simulink model "buck_hysteresis"  (Simulink 8.9)
settings: Solver=ode45  StartTime=0.0  StopTime=Tmax  RelTol=1e-3  EnableMultiTasking=on
values from neighbouring files (symbols this model uses):
  a00c = sys(1).Ac(1,1)    [buck_parameters.m]
  a00d = sys(1).Ad(1,1)    [buck_parameters.m]
  a00o = sys(1).Ao(1,1)    [buck_parameters.m]
  a01c = sys(1).Ac(1,2)    [buck_parameters.m]
  a01d = sys(1).Ad(1,2)    [buck_parameters.m]
  a01o = sys(1).Ao(1,2)    [buck_parameters.m]
  a10c = sys(1).Ac(2,1)    [buck_parameters.m]
  a10d = sys(1).Ad(2,1)    [buck_parameters.m]
  a10o = sys(1).Ao(2,1)    [buck_parameters.m]
  a11c = sys(1).Ac(2,2)    [buck_parameters.m]
  a11d = sys(1).Ad(2,2)    [buck_parameters.m]
  a11o = sys(1).Ao(2,2)    [buck_parameters.m]
  b0c = sys(1).Bc(1)    [buck_parameters.m]
  b0d = sys(1).Bd(1)    [buck_parameters.m]
  b0o = sys(1).Bo(1)    [buck_parameters.m]
  b1c = sys(1).Bc(2)    [buck_parameters.m]
  b1d = sys(1).Bd(2)    [buck_parameters.m]
  b1o = sys(1).Bo(2)    [buck_parameters.m]
  i0 = 0    [buck_parameters.m]
  v0 = 0    [buck_parameters.m]
  Vref = 12    [buck_parameters.m]
  Vtol = Vref/120    (= 0.1)    [buck_parameters.m]
settings Model: Creator=Omar Ali Beg  LastModifiedBy=LuanNguyen
settings OptimizationCC: ExpressionDepthLimit=2147483647
settings DebuggingCC: MaxConsecutiveZCsMsg=none  MultiTaskDSMMsg=warning  MultiTaskCondExecSysMsg=none  FcnCallInpInsideContextMsg=error  StrictBusMsg=None
settings GRTTargetCC: CombineOutputUpdateFcns=on  GRTInterface=off

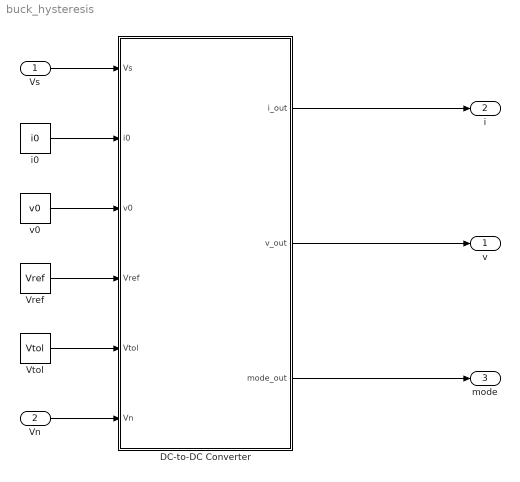
== system buck_hysteresis ==
  Vs : Inport
  Vn : Inport  Port=2
  DC-to-DC Converter : Stateflow chart  TreatAsAtomicUnit=on
  Vref : Constant  Value=Vref
  Vtol : Constant  Value=Vtol
  i0 : Constant  Value=i0
  v0 : Constant  Value=v0
  v : Outport
  i : Outport  Port=2
  mode : Outport  Port=3
  wires:
  DC-to-DC Converter/2(v_out) -> v/1
  Vs/1 -> DC-to-DC Converter/1(Vs)
  i0/1 -> DC-to-DC Converter/2(i0)
  v0/1 -> DC-to-DC Converter/3(v0)
  Vref/1 -> DC-to-DC Converter/4(Vref)
  DC-to-DC Converter/3(mode_out) -> mode/1
  Vtol/1 -> DC-to-DC Converter/5(Vtol)
  DC-to-DC Converter/1(i_out) -> i/1
  Vn/1 -> DC-to-DC Converter/6(Vn)

== stateflow chart DC-to-DC Converter ==
  settings: updateMethod=CONTINUOUS
  state Discontinuous
    du:
    i_dot = a00d*i+a01d*v+b0d*(Vs+Vn);
    v_dot = a10d*i+a11d*v+b1d*(Vs+Vn);
    t_dot = 1;
    i_out =i;
    v_out = v;
    mode_out=3;
  state Charging
    du:
    i_dot = a00c*i+a01c*v+b0c*(Vs+Vn);
    v_dot = a10c*i+a11c*v+b1c*(Vs+Vn);
    t_dot = 1;
    i_out = i;
    v_out = v;
    mode_out=2;
  state Discharging
    du:
    i_dot = a00o*i+a01o*v+b0o*(Vs+Vn);
    v_dot = a10o*i+a11o*v+b1o*(Vs+Vn);
    t_dot = 1;
    i_out = i;
    v_out = v;
    mode_out=1;
  Discontinuous -> Charging : [v <= Vref-Vtol]
  Discharging -> Discontinuous [order 1] : [i <= 0]
  (default) -> Charging : {i = i0;
      | v = v0;}
  Charging -> Discharging : [v >= Vref+Vtol]
  Discharging -> Charging [order 2] : [v <= Vref-Vtol]
  data: t local double; i_out output double; v_out output double; i local double; a00o local double; Vs input double =120; a01o local double; a10o local double; a11o local double; a00c local double; a01c local double; a10c local double; a11c local double; b0o local double; b1o local double; b0c local double; b1c local double; v local double; i0 input double; v0 input double; a01d local double; a10d local double; a11d local double; a00d local double; b0d local double; b1d local double; Vref input double =120; mode_out output double; Vtol input double =120; Vn input double =120
  data t settings: updateMethod=SF_CONTINUOUS_TIME_DATA
  data i settings: updateMethod=SF_CONTINUOUS_TIME_DATA
  data v settings: updateMethod=SF_CONTINUOUS_TIME_DATA
  data Vtol settings: description=Voltage tolerance (e.g., Vref / 100 is +/- 1% voltage ripple)
